simulink model "choir_sim"  (R2026b)
settings: Solver=FixedStepDiscrete  StopTime=8.5125000000000011
settings Model: Creator=rachnap  LastModifiedBy=rachnap

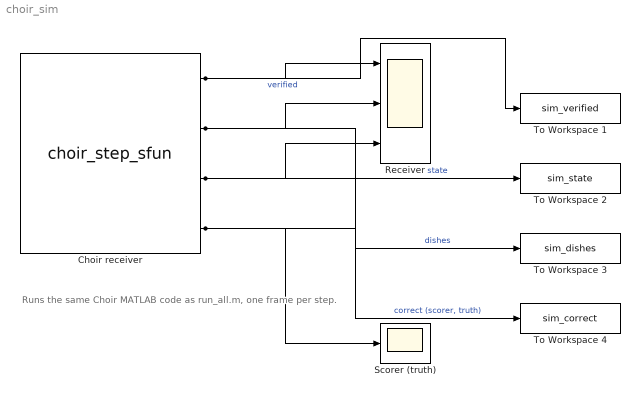
== system choir_sim ==
  note: Runs the same Choir MATLAB code as run_all.m, one frame per step.
  Choir receiver : M-S-Function  FunctionName=choir_step_sfun
  Receiver : Scope  NumInputPorts=3
  Scorer (truth) : Scope
  To Workspace 1 : ToWorkspace  VariableName=sim_verified  SaveFormat=Timeseries  SampleTime=-1
  To Workspace 2 : ToWorkspace  VariableName=sim_state  SaveFormat=Timeseries  SampleTime=-1
  To Workspace 3 : ToWorkspace  VariableName=sim_dishes  SaveFormat=Timeseries  SampleTime=-1
  To Workspace 4 : ToWorkspace  VariableName=sim_correct  SaveFormat=Timeseries  SampleTime=-1
  wires:
  Choir receiver/1 -> Receiver/1, To Workspace 1/1  "verified"
  Choir receiver/2 -> Receiver/2, To Workspace 2/1  "state"
  Choir receiver/3 -> Receiver/3, To Workspace 3/1  "dishes"
  Choir receiver/4 -> Scorer (truth)/1, To Workspace 4/1  "correct (scorer, truth)"
